simulink model "BDrivetrainCoolingOn"  (R2024b)
settings: configuration reference "STM32H7_Config" (kept outside this file)
libraries: simulink x3
settings Model: DataDictionary=Master_Dictionary.sldd  EnableAccessToBaseWorkspace=off  Creator=torni  LastModifiedBy=Will
settings ConfigSetRef: SourceName=STM32H7_Config

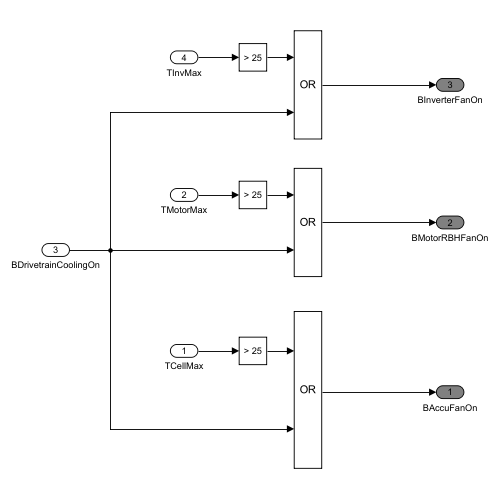
[thumbnail: Simulink's stored preview of the top-level diagram]
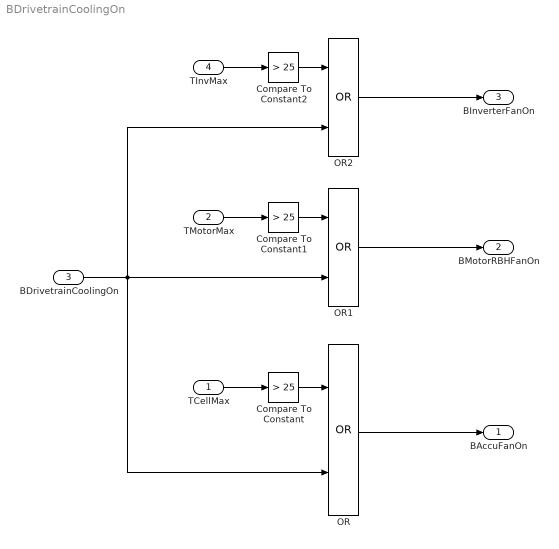
== system BDrivetrainCoolingOn ==
  TCellMax : Inport  OutDataTypeStr=double
  TMotorMax : Inport  Port=2  OutDataTypeStr=double
  BDrivetrainCoolingOn : Inport  Port=3  OutDataTypeStr=boolean
  TInvMax : Inport  Port=4  OutDataTypeStr=double
  Compare To Constant : simulink/Logic and Bit Operations/Compare To Constant  relop=>  const=25  OutDataTypeStr=boolean
  Compare To Constant1 : simulink/Logic and Bit Operations/Compare To Constant  relop=>  const=25  OutDataTypeStr=boolean
  Compare To Constant2 : simulink/Logic and Bit Operations/Compare To Constant  relop=>  const=25  OutDataTypeStr=boolean
  OR : Logic  Operator=OR  AllPortsSameDT=off  OutDataTypeStr=boolean
  OR1 : Logic  Operator=OR  AllPortsSameDT=off  OutDataTypeStr=boolean
  OR2 : Logic  Operator=OR  AllPortsSameDT=off  OutDataTypeStr=boolean
  BAccuFanOn : Outport  OutDataTypeStr=boolean  VectorParamsAs1DForOutWhenUnconnected=off
  BMotorRBHFanOn : Outport  Port=2  OutDataTypeStr=boolean  VectorParamsAs1DForOutWhenUnconnected=off
  BInverterFanOn : Outport  Port=3  OutDataTypeStr=boolean  VectorParamsAs1DForOutWhenUnconnected=off
  wires:
  TCellMax/1 -> Compare To Constant/1
  BDrivetrainCoolingOn/1 -> OR/2, OR1/2, OR2/2
  OR1/1 -> BMotorRBHFanOn/1
  Compare To Constant2/1 -> OR2/1
  Compare To Constant1/1 -> OR1/1
  TInvMax/1 -> Compare To Constant2/1
  OR2/1 -> BInverterFanOn/1
  TMotorMax/1 -> Compare To Constant1/1
  OR/1 -> BAccuFanOn/1
  Compare To Constant/1 -> OR/1
